simulink model "BSA"  (R2018a)
settings: Solver=ode1  StartTime=0.0  StopTime=Inf  FixedStep=0.001  RelTol=1e-3
PostLoadFcn:
  | , if any(exist('dsrtsu_mdlpostloadfcn', 'file') == [2, 3, 6]), try dsrtsu_mdlpostloadfcn('Execute', bdroot); catch fprintf('Error in PostLoadFcn (dsrtsu_mdlpostloadfcn) for model "%s":\n %s\n', bdroot, lasterr); end, end,
Description:
  | Standard RTI1007 template.
  | Supported MATLAB version:  R2018b.
settings Model: Tag=RTI1007  DSRTSU_INTERNAL_RTI_VER=530  DSRTSU_INTERNAL_RTI_TYPE=rti1007  RTICANMMDATA=struct('GeneralSetupData',struct('modelroot','Z:\public\Transfer\Mueller\DOB','generalsettings',struct('filesettings',struct('destfolder',struct('Name','RTICANMM_FILES','Check',1),'buildfolder',struct('Name','.','Check',1),'AbsDestfolder',struct('Name','Z:\public\Transfer\Mueller\DOB\RTICANMM_FILES'),'AbsBuildfolder',struct('Name','Z:\public\Transfer\Mueller\DOB'))),'options',struct('addpaths',1,'rmpaths',1,'addtrcexclusion',logical(1),'cannavigator',struct('checkmonitoring',0),'show_usrtrc',0,'use_usrtrc',0),'advanced',struct('options',ones(1,100)),'MPSetup',{{}},'RTI',struct('Type','RTI1007','Ver','7.11','Date','02-Nov-2018'),'modelname','seven_Dof','block','seven_Dof'))  DSRTSU_INTERNAL_RTIFPGA=120  Creator=User  LastModifiedBy=Müller
settings OptimizationCC: BlockReduction=off  OptimizeBlockIOStorage=off  BufferReuse=off  GlobalBufferReuse=off  ExpressionFolding=off  LocalBlockOutputs=off  OptimizeDataStoreBuffers=off  BusAssignmentInplaceUpdate=off
settings HardwareCC: ProdBitPerPointer=32  ProdBitPerSizeT=32  ProdBitPerPtrDiffT=32  ProdLargestAtomicInteger=Integer  ProdEndianess=BigEndian  ProdWordSize=32  ProdHWDeviceType=Custom Processor->Custom  TargetIntDivRoundTo=Zero  TargetEndianess=BigEndian  TargetHWDeviceType=Custom Processor->Custom
settings SFSimCC: MATLABDynamicMemAlloc=off
settings RTWCC: SystemTargetFile=rti1007.tlc  MakeCommand=make_rti  TemplateMakefile=rti1007.tmf  Description=dSPACE DS1007 Hardware Platform
settings CodeAppCC: StateflowObjectComments=on
settings STFCustomTargetCC: ParMdlRefBuildCompliant=on  MatFileLogging=on  GRTInterface=off  SystemTargetFile=rti1007.tlc
settings GRTTargetCC: TargetLangStandard=C89/C90 (ANSI)  CompOptLevelCompliant=off  ConcurrentExecutionCompliant=off  CombineOutputUpdateFcns=off  CPPClassGenCompliant=off  UseToolchainInfoCompliant=off
settings ConfigComp: CovMetricSettings=dswe

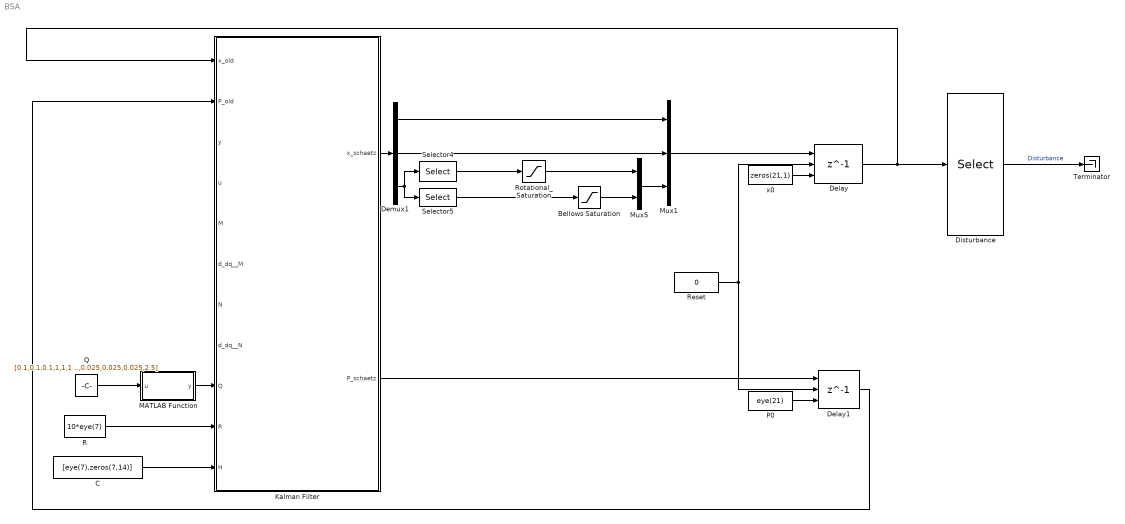
== system BSA ==
  Bellows Saturation : Saturate  UpperLimit=1  LowerLimit=-1
  C : Constant  Value=[eye(7),zeros(7,14)]
  Delay : Delay  DelayLength=1  InitialConditionSource=Input port  ExternalReset=Rising
      settings: InputPortMap=u0,r5,p4
  Delay1 : Delay  DelayLength=1  InitialConditionSource=Input port  ExternalReset=Rising
      settings: InputPortMap=u0,r5,p4
  Demux1 : Demux  Outputs=3
  Disturbance : Selector  InputPortWidth=21  IndexOptions=Index vector (dialog)  Indices=15:21  OutputSizes=1
  Kalman Filter : MATLAB Function  TreatAsAtomicUnit=on
  MATLAB Function : MATLAB Function  TreatAsAtomicUnit=on
  Mux1 : Mux  Inputs=3
  Mux5 : Mux  Inputs=2
  P0 : Constant  Value=eye(21)
  Q : Constant  Value=[0.1,0.1,0.1,1,1,1,0.01,0.001,0.001,0.001,1000,1000,1000,0.1,0.25,0.25,0.25,0.025,0.025,0.025,2.5]
  R : Constant  Value=10*eye(7)
  Reset : Constant  Value=0
  Rotational_Saturation : Saturate  UpperLimit=2  LowerLimit=-2
  Selector4 : Selector  InputPortWidth=7  IndexOptions=Index vector (dialog)  Indices=[1:3]  OutputSizes=1
  Selector5 : Selector  InputPortWidth=7  IndexOptions=Index vector (dialog)  Indices=[4:7]  OutputSizes=1
  Terminator : Terminator
  x0 : Constant  Value=zeros(21,1)
  wires:
  Demux1/1 -> Mux1/1
  Kalman Filter/1(x_schaetz) -> Demux1/1
  Reset/1 -> Delay1/2, Delay/2
  x0/1 -> Delay/3
  Rotational_Saturation/1 -> Mux5/1
  Demux1/3 -> Selector4/1, Selector5/1
  Delay/1 -> Disturbance/1, Kalman Filter/1(x_old)
  Bellows Saturation/1 -> Mux5/2
  Delay1/1 -> Kalman Filter/2(P_old)
  Demux1/2 -> Mux1/2
  Selector5/1 -> Bellows Saturation/1
  Selector4/1 -> Rotational_Saturation/1
  Mux5/1 -> Mux1/3
  Mux1/1 -> Delay/1
  P0/1 -> Delay1/3
  Kalman Filter/2(P_schaetz) -> Delay1/1
  C/1 -> Kalman Filter/11(H)
  R/1 -> Kalman Filter/10(R)
  MATLAB Function/1(y) -> Kalman Filter/9(Q)
  Q/1 -> MATLAB Function/1(u)
  Disturbance/1 -> Terminator/1  "Disturbance"

== matlab function BSA/MATLAB Function ==
  data: u input; y output
function y = makeDiag(u)

y = diag(u);

== matlab function BSA/Kalman Filter ==
  data: x_old input; P_old input; y input; u input; x_schaetz output; M input; d_dq__M input; N input; d_dq__N input; Q input; R input; P_schaetz output; H input
function [x_schaetz,P_schaetz] = fcn(x_old,P_old,y,u,M,d_dq__M,N,d_dq__N,Q,R,H)%
%% @author daniel.mueller@isys.uni-stuttgart.de
% Inputs:   x_old - last step observer state
%            P_old - Covariance Noise
%            y - Measurement
%            u - Mechanical input, i.e. tau in the paper
%            M - Intertia matrix
%            d_dq__M - derivative of Intertia matrix
%            N - Gravitational Force
%            d_dq__N - derivative of Gravitational Froce
%            Q - System noise
%            R - Measurment noise
%            H - Derivative of the output equation h(x), note that it is
%                g(x) in the paper
% Implementation and convetnion of the EKF according to Wikipedia 
%                    (https://en.wikipedia.org/wiki/Extended_Kalman_filter)

%Sample Time
dt = 1e-3;
%System equation
f = [x_old(8:14);
    M\(u-N+x_old(15:21));
    zeros(7,1)];

%Derivative of System equation
F = zeros(21,21);
F_int = [eye(7),zeros(7,14);
    zeros(7), eye(7), zeros(7);
    zeros(7,14), eye(7)];
% P = eye(12); %Initial value
for ii = 1:7
    F(8:14,ii) = M\((d_dq__M(:,:,ii)/M)*(u-N+x_old(15:21))-d_dq__N(:,ii));
end
F(1:7,8:14) = eye(7);
F(8:14,15:21) = M\eye(7);
F(:,:) = dt*(F(:,:))+F_int;

%% Prediction
x_pred =  x_old + dt*f;
P_pred = F*P_old*F' + Q;
%% Update
S = R + H*P_pred*H';
K = P_pred*H'/S;
P_schaetz = (eye(21)-K*H)*P_pred;
x_schaetz = x_pred + K*(y-H*x_pred);

end
